simulink model "Sim_app"  (R2023b)
settings: Solver=ode1  StartTime=0.0  StopTime=inf  FixedStep=0.01  RelTol=1e-3
undefined symbols (not defined in the file or in its folder): T1_high, T1_low, T2_high, T2_low
libraries: simulink x2, qbmove_library x2, dspstat3 x1, QB_pacer_lib x1
settings Model: Creator=ilari  LastModifiedBy=ilari
settings DataIOCC: OutputSaveName=out

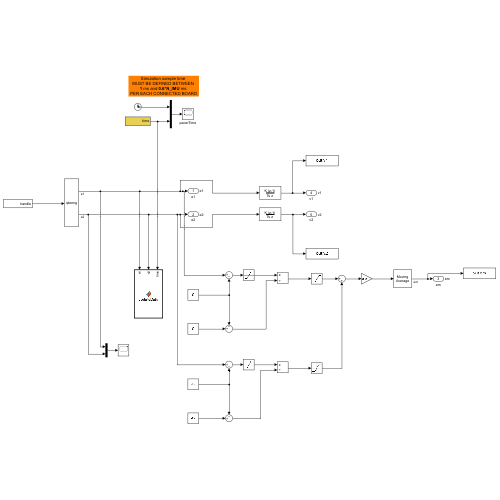
[thumbnail: Simulink's stored preview of the top-level diagram]
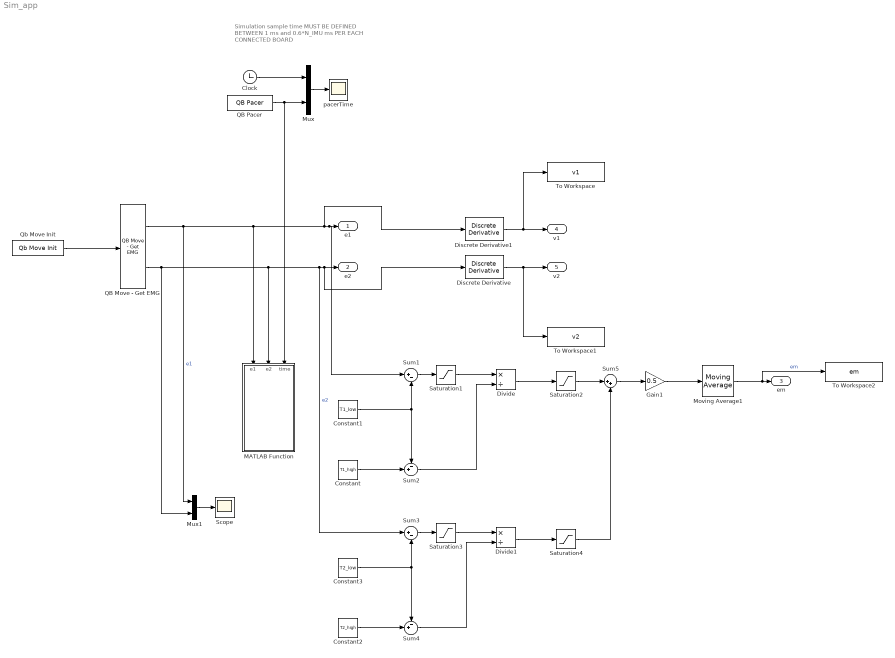
== system Sim_app ==
  note: Simulation sample time
      | MUST BE DEFINED BETWEEN
      | 1 ms and 0.6*N_IMU ms
      | PER EACH CONNECTED BOARD
  Clock : Clock
  Constant : Constant  Value=T1_high
  Constant1 : Constant  Value=T1_low
  Constant2 : Constant  Value=T2_high
  Constant3 : Constant  Value=T2_low
  Discrete Derivative : simulink/Discrete/Discrete Derivative  gainval=1.0  ICPrevScaledInput=0.0  OutMin=[]  OutMax=[]  OutDataType=fixdt(1, 16)  OutScaling=2^-10  DoSatur=off
  Discrete Derivative1 : simulink/Discrete/Discrete Derivative  gainval=1.0  ICPrevScaledInput=0.0  OutMin=[]  OutMax=[]  OutDataType=fixdt(1, 16)  OutScaling=2^-10  DoSatur=off
  Divide : Product  Inputs=*/
  Divide1 : Product  Inputs=*/
  Gain1 : Gain  Gain=0.5
  MATLAB Function : MATLAB Function  TreatAsAtomicUnit=on
  Moving Average1 : dspstat3/Moving Average  Method=Sliding window  ForgettingFactorPort=off  SpecifyWindowLength=on  WindowLength=5  OverlapLength=4  AllowArbitraryInputLength=off  ForgettingFactor=0.9  SimulateUsing=Code generation
  Mux : Mux  Inputs=2
  Mux1 : Mux  Inputs=2
  QB Move - Get EMG : qbmove_library/QB Move - Get EMG  ID=10  DAISY_CHAINING=off
      settings: SourceProductName=Qb Move Library
  QB Pacer : QB_pacer_lib/QB Pacer  simTimePerRealTime=1
      settings: SourceProductName=QB Pacer
  Qb Move Init : qbmove_library/Qb Move Init  NUMBER_OF_COM='COM7'  BAUD_RATE_COM=2000000
      settings: SourceProductName=Qb Move Library
  Saturation1 : Saturate  UpperLimit=1024  LowerLimit=0
  Saturation2 : Saturate  UpperLimit=1  LowerLimit=0
  Saturation3 : Saturate  UpperLimit=1024  LowerLimit=0
  Saturation4 : Saturate  UpperLimit=1  LowerLimit=0
  Scope : Scope
  Sum1 : Sum  Inputs=|+-
  Sum2 : Sum  Inputs=-+|
  Sum3 : Sum  Inputs=|+-
  Sum4 : Sum  Inputs=-+|
  Sum5 : Sum  Inputs=|++
  To Workspace : ToWorkspace  VariableName=v1  SaveFormat=Timeseries  SampleTime=-1
  To Workspace1 : ToWorkspace  VariableName=v2  SaveFormat=Timeseries  SampleTime=-1
  To Workspace2 : ToWorkspace  VariableName=em  SaveFormat=Timeseries  SampleTime=-1
  pacerTime : Scope
  e1 : Outport  SignalName=e1
  e2 : Outport  Port=2  SignalName=e2
  em : Outport  Port=3  SignalName=em
  v1 : Outport  Port=4  SignalName=v1
  v2 : Outport  Port=5  SignalName=v2
  wires:
  Mux/1 -> pacerTime/1
  Clock/1 -> Mux/1
  Qb Move Init/1 -> QB Move - Get EMG/1
  QB Move - Get EMG/1 -> Mux1/1, Discrete Derivative1/1, Sum1/1, e1/1, MATLAB Function/1(e1)  "e1"
  QB Move - Get EMG/2 -> Mux1/2, Sum3/1, Discrete Derivative/1, e2/1, MATLAB Function/2(e2)  "e2"
  Constant/1 -> Sum2/2
  Constant1/1 -> Sum2/1, Sum1/2
  Saturation3/1 -> Divide1/1
  Sum3/1 -> Saturation3/1
  Constant3/1 -> Sum4/1, Sum3/2
  Sum4/1 -> Divide1/2
  Divide1/1 -> Saturation4/1
  Saturation1/1 -> Divide/1
  Sum2/1 -> Divide/2
  Constant2/1 -> Sum4/2
  Sum5/1 -> Gain1/1
  Sum1/1 -> Saturation1/1
  Saturation2/1 -> Sum5/1
  Moving Average1/1 -> To Workspace2/1, em/1  "em"
  Saturation4/1 -> Sum5/2
  Gain1/1 -> Moving Average1/1
  Divide/1 -> Saturation2/1
  Discrete Derivative/1 -> To Workspace1/1, v2/1
  Discrete Derivative1/1 -> To Workspace/1, v1/1
  QB Pacer/1 -> Mux/2, MATLAB Function/3(time)
  Mux1/1 -> Scope/1

== matlab function Sim_app/MATLAB Function ==
  data: e1 input; e2 input; time input
function updateData(e1, e2, time)

    assignin('base', 'e1_Live', e1);
    assignin('base', 'e2_Live', e2);
    assignin('base', 'Time_Live', time);
    
    % evalin('base', sprintf('Time_Live(end+1) = %f', time))
    % evalin('base', sprintf('e1_Live(end+1) = %f', e1))
    % evalin('base', sprintf('e2_Live(end+1) = %f', e2))


end
